simulink model "simulacionfinal"  (R2014a)
settings: Solver=ode3  StartTime=0.0  StopTime=40  FixedStep=0.01  RelTol=1e-12
values from neighbouring files (symbols this model uses):
  m = [1 t0 (t0)^2 (t0)^3;0 1 (2*(t0)^2) (3*(t0)^2);1 tf (tf)^2 (tf)^3;0 1 (2*(tf)^2) (3*(tf)^2)]    [ControlCinematico.m]    (also in untitled3.m = [1 0 0 0 0 0;0 1 0 0 0 0;0 0 2 0 0 0;1 tf tf^2 tf^3 tf^4 tf^)
libraries: mblibv1 x15
settings Model: Creator=sebastian  LastModifiedBy=root
settings DataIOCC: SignalLoggingSaveFormat=ModelDataLogs
settings DebuggingCC: UnderspecifiedInitializationDetection=Classic  MultiTaskDSMMsg=warning  MultiTaskCondExecSysMsg=none  StateNameClashWarn=warning
settings RTWCC: IncludeERTFirstTime=on
settings SimMechanicsCC: VisOnUpdateDiagram=on  VisDuringSimulation=on

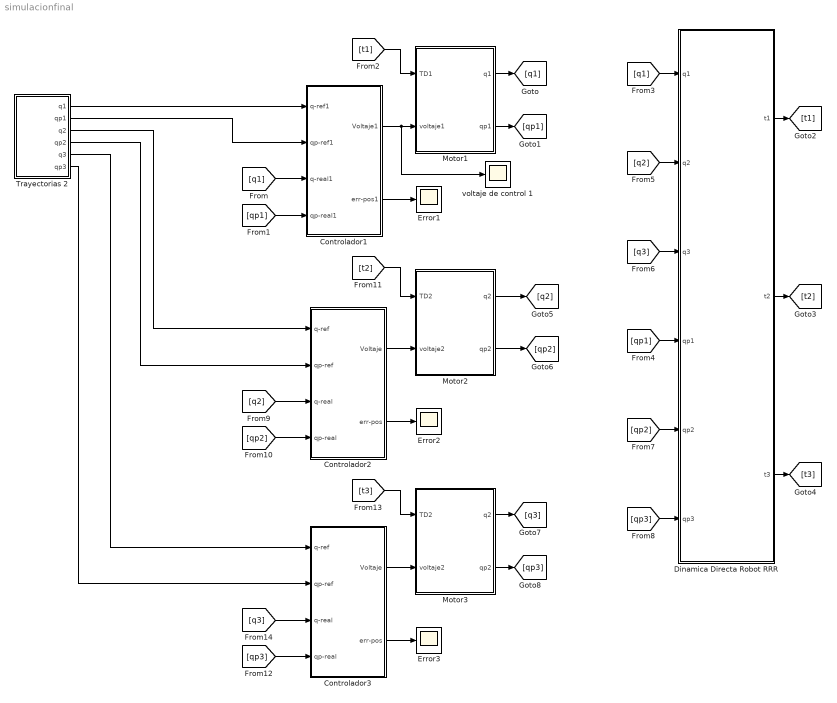
== system simulacionfinal ==
  Controlador1 : Subsystem
  Controlador2 : Subsystem
  Controlador3 : Subsystem
  Dinamica Directa Robot RRR : Subsystem
  Error1 : Scope
      settings: TimeRange=0.000199999999999978  YMin=-470000  YMax=-455000  SaveName=ScopeData4
  Error2 : Scope
      settings: YMin=0.3178  YMax=0.3188
  Error3 : Scope
      settings: YMin=0.675  YMax=1  SaveName=ScopeData5
  Motor1 : Subsystem
  Motor2 : Subsystem
  Motor3 : Subsystem
  Trayectorias 2 : Subsystem
  voltaje de control 1 : Scope
      settings: YMin=-1.5  YMax=1.25  SaveName=ScopeData12
  wires:
  Controlador1/1(Voltaje1) -> voltaje de control 1/1, Motor1/2(voltaje1)
  Controlador1/2(err-pos1) -> Error1/1
  Motor1/1(q1) -> [q1]
  Motor1/2(qp1) -> [qp1]
  Dinamica Directa Robot RRR/1(t1) -> [t1]
  [q1] -> Controlador1/3(q-real1)
  [qp1] -> Controlador1/4(qp-real1)
  [q1] -> Dinamica Directa Robot RRR/1(q1)
  [qp1] -> Dinamica Directa Robot RRR/4(qp1)
  [q2] -> Dinamica Directa Robot RRR/2(q2)
  [q3] -> Dinamica Directa Robot RRR/3(q3)
  [qp2] -> Dinamica Directa Robot RRR/5(qp2)
  [qp3] -> Dinamica Directa Robot RRR/6(qp3)
  Dinamica Directa Robot RRR/2(t2) -> [t2]
  Dinamica Directa Robot RRR/3(t3) -> [t3]
  Controlador2/1(Voltaje) -> Motor2/2(voltaje2)
  Controlador2/2(err-pos) -> Error2/1
  [q2] -> Controlador2/3(q-real)
  [qp2] -> Controlador2/4(qp-real)
  Controlador3/1(Voltaje) -> Motor3/2(voltaje2)
  Controlador3/2(err-pos) -> Error3/1
  Motor3/1(q2) -> [q3]
  Motor3/2(qp2) -> [qp3]
  [q3] -> Controlador3/3(q-real)
  [qp3] -> Controlador3/4(qp-real)
  Motor2/1(q2) -> [q2]
  Motor2/2(qp2) -> [qp2]
  Trayectorias 2/1(q1) -> Controlador1/1(q-ref1)
  Trayectorias 2/2(qp1) -> Controlador1/2(qp-ref1)
  Trayectorias 2/3(q2) -> Controlador2/1(q-ref)
  Trayectorias 2/4(qp2) -> Controlador2/2(qp-ref)
  Trayectorias 2/5(q3) -> Controlador3/1(q-ref)
  Trayectorias 2/6(qp3) -> Controlador3/2(qp-ref)
  [t1] -> Motor1/1(TD1)
  [t2] -> Motor2/1(TD2)
  [t3] -> Motor3/1(TD2)

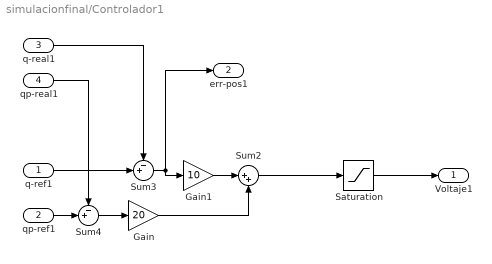
== system simulacionfinal/Controlador1 ==
  q-ref1 : Inport
  qp-ref1 : Inport  Port=2
  q-real1 : Inport  Port=3
  qp-real1 : Inport  Port=4
  Gain : Gain  Gain=20
  Gain1 : Gain  Gain=10
  Saturation : Saturate  UpperLimit=1.5  LowerLimit=-1.5
  Sum2 : Sum  Inputs=|++
  Sum3 : Sum  Inputs=-+|
  Sum4 : Sum  Inputs=-+|
  Voltaje1 : Outport
  err-pos1 : Outport  Port=2
  wires:
  Gain1/1 -> Sum2/1
  Gain/1 -> Sum2/2
  Sum4/1 -> Gain/1
  Sum2/1 -> Saturation/1
  q-ref1/1 -> Sum3/2
  qp-ref1/1 -> Sum4/2
  q-real1/1 -> Sum3/1
  qp-real1/1 -> Sum4/1
  Sum3/1 -> Gain1/1, err-pos1/1
  Saturation/1 -> Voltaje1/1

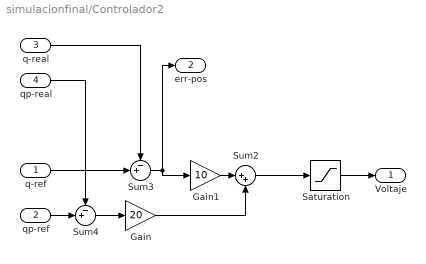
== system simulacionfinal/Controlador2 ==
  q-ref : Inport
  qp-ref : Inport  Port=2
  q-real : Inport  Port=3
  qp-real : Inport  Port=4
  Gain : Gain  Gain=20
  Gain1 : Gain  Gain=10
  Saturation : Saturate  UpperLimit=1.5  LowerLimit=-1.5
  Sum2 : Sum  Inputs=|++
  Sum3 : Sum  Inputs=-+|
  Sum4 : Sum  Inputs=-+|
  Voltaje : Outport
  err-pos : Outport  Port=2
  wires:
  Gain1/1 -> Sum2/1
  Gain/1 -> Sum2/2
  Sum4/1 -> Gain/1
  Sum2/1 -> Saturation/1
  q-ref/1 -> Sum3/2
  qp-ref/1 -> Sum4/2
  q-real/1 -> Sum3/1
  qp-real/1 -> Sum4/1
  Sum3/1 -> Gain1/1, err-pos/1
  Saturation/1 -> Voltaje/1

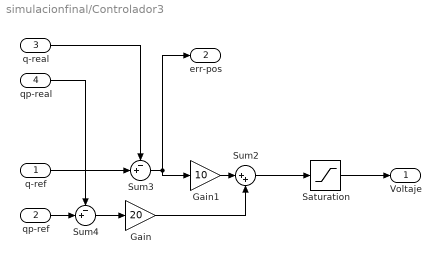
== system simulacionfinal/Controlador3 ==
  q-ref : Inport
  qp-ref : Inport  Port=2
  q-real : Inport  Port=3
  qp-real : Inport  Port=4
  Gain : Gain  Gain=20
  Gain1 : Gain  Gain=10
  Saturation : Saturate  UpperLimit=1.5  LowerLimit=-1.5
  Sum2 : Sum  Inputs=|++
  Sum3 : Sum  Inputs=-+|
  Sum4 : Sum  Inputs=-+|
  Voltaje : Outport
  err-pos : Outport  Port=2
  wires:
  Gain1/1 -> Sum2/1
  Gain/1 -> Sum2/2
  Sum4/1 -> Gain/1
  Sum2/1 -> Saturation/1
  q-ref/1 -> Sum3/2
  qp-ref/1 -> Sum4/2
  q-real/1 -> Sum3/1
  qp-real/1 -> Sum4/1
  Sum3/1 -> Gain1/1, err-pos/1
  Saturation/1 -> Voltaje/1

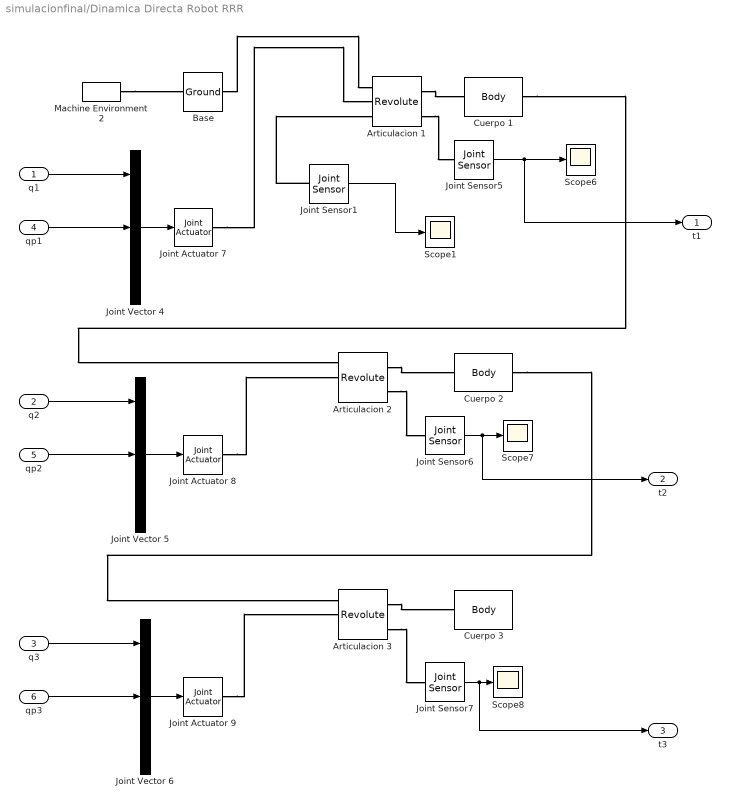
== system simulacionfinal/Dinamica Directa Robot RRR ==
  q1 : Inport
  q2 : Inport  Port=2
  q3 : Inport  Port=3
  qp1 : Inport  Port=4
  qp2 : Inport  Port=5
  qp3 : Inport  Port=6
  Articulacion 1 : mblibv1/Joints/Revolute  LConnTagsString=__newl0|SA1|SA2  RConnTagsString=__newr0|SA1  UpdateFromCAD=off  NumSAPorts=3  CutJoint=off  MarkAsCut=off  Primitives=prismatic  PrimitiveProps=R1$World$[0 0 1]$revolute  DialogClass=JointBlock  R1Axis=[0 0 1]
  Articulacion 2 : mblibv1/Joints/Revolute  LConnTagsString=__newl0|SA1|SA2  RConnTagsString=__newr0|SA1  UpdateFromCAD=off  NumSAPorts=3  CutJoint=off  MarkAsCut=off  Primitives=prismatic  PrimitiveProps=R1$World$[0 0 1]$revolute  DialogClass=JointBlock  R1Axis=[0 0 1]
  Articulacion 3 : mblibv1/Joints/Revolute  LConnTagsString=__newl0|SA1|SA2  RConnTagsString=__newr0|SA1  UpdateFromCAD=off  NumSAPorts=3  CutJoint=off  MarkAsCut=off  Primitives=prismatic  PrimitiveProps=R1$World$[0 0 1]$revolute  DialogClass=JointBlock  R1Axis=[0 0 1]
  Base : mblibv1/Bodies/Ground  UpdateFromCAD=off  LeftPortType=env  RightPortType=workingframe  PhysicalDomain=Mechanical  DialogClass=GroundBlock  CoordPosition=[0 0 0]  CoordPositionUnits=m  StateVectorMgrId=0  MachineId=[1 0]  ShowEnvPort=on  ParameterChecksum=[135980113, 3777956771, 1224883924, 2878565293]  TopologyChecksum=[1058938833, 390769295, 436021046, 484204497]
  Cuerpo 1 : mblibv1/Bodies/Body  LConnTagsString=CS1  RConnTagsString=CS2  UpdateFromCAD=off  DialogClass=MechanicalBodyBlock  Mass=1  MassUnits=kg  InertiaUnits=kg*m^2  Inertia=[0 0 0;0 0 0;0 0 33.3333]  Shape=Cylinder  ShapeDims=[1 1]  ShapeUnits=m  ShapeUse=false  Density=1  DensityUnits=kg/m^3  DensityUse=false  GraphicsMode=MACHINE_DEFAULT  BodyColorSelMode=COLORPALETTE  BodyColor=[0 1 0]  AttachedToCS=CG  CG=Left$CG$[0 10 0]$WORLD$WORLD$m$[0 0 0]$Euler X-Y-Z$deg$WORLD$false$none  WorkingFrames=Left$CS1$[0 0 0]$World$World$m$[0 0 0]$Euler X-Y-Z$deg$WORLD$true$none#Right$CS2$[0 20 0]$World$World$m$[0 0 0]$Euler X-Y-Z$deg$WORLD$true$none  CGPos=[0 10 0]  CGRot=[0 0 0]  CS0Pos=[]  CS0Rot=[]  CS1Pos=[0 0 0]  CS1Rot=[0 0 0]  CS2Pos=[0 20 0]  CS2Rot=[0 0 0]  CS3Pos=[]  CS3Rot=[]  CS4Pos=[]  CS4Rot=[]  CS5Pos=[]  CS5Rot=[]  CS6Pos=[]  CS6Rot=[]  CS7Pos=[]  CS7Rot=[]  CS8Pos=[]  CS8Rot=[]  CS9Pos=[]  CS9Rot=[]  CS10Pos=[]  CS10Rot=[]  CS11Pos=[]  CS11Rot=[]  CS12Pos=[]  CS12Rot=[]  CS13Pos=[]  CS13Rot=[]  CS14Pos=[]  CS14Rot=[]  CS15Pos=[]  CS15Rot=[]  CS16Pos=[]  CS16Rot=[]  CS17Pos=[]  CS17Rot=[]  CS18Pos=[]  CS18Rot=[]  CS19Pos=[]  CS19Rot=[]  CS20Pos=[]  CS20Rot=[]
  Cuerpo 2 : mblibv1/Bodies/Body  LConnTagsString=CS1  RConnTagsString=CS2  UpdateFromCAD=off  DialogClass=MechanicalBodyBlock  Mass=1  MassUnits=kg  InertiaUnits=kg*m^2  Inertia=[0 0 0;0 0 0;0 0 33.3333]  Shape=Cylinder  ShapeDims=[1 1]  ShapeUnits=m  ShapeUse=false  Density=1  DensityUnits=kg/m^3  DensityUse=false  GraphicsMode=MACHINE_DEFAULT  BodyColorSelMode=COLORPALETTE  BodyColor=[0 1 0]  AttachedToCS=CG  CG=Left$CG$[10 20 0]$WORLD$WORLD$m$[0 0 0]$Euler X-Y-Z$deg$WORLD$false$none  WorkingFrames=Left$CS1$[0 20 0]$World$World$m$[0 0 0]$Euler X-Y-Z$deg$WORLD$true$none#Right$CS2$[20 20 0]$World$World$m$[0 0 0]$Euler X-Y-Z$deg$WORLD$true$none  CGPos=[10 20 0]  CGRot=[0 0 0]  CS0Pos=[]  CS0Rot=[]  CS1Pos=[0 20 0]  CS1Rot=[0 0 0]  CS2Pos=[20 20 0]  CS2Rot=[0 0 0]  CS3Pos=[]  CS3Rot=[]  CS4Pos=[]  CS4Rot=[]  CS5Pos=[]  CS5Rot=[]  CS6Pos=[]  CS6Rot=[]  CS7Pos=[]  CS7Rot=[]  CS8Pos=[]  CS8Rot=[]  CS9Pos=[]  CS9Rot=[]  CS10Pos=[]  CS10Rot=[]  CS11Pos=[]  CS11Rot=[]  CS12Pos=[]  CS12Rot=[]  CS13Pos=[]  CS13Rot=[]  CS14Pos=[]  CS14Rot=[]  CS15Pos=[]  CS15Rot=[]  CS16Pos=[]  CS16Rot=[]  CS17Pos=[]  CS17Rot=[]  CS18Pos=[]  CS18Rot=[]  CS19Pos=[]  CS19Rot=[]  CS20Pos=[]  CS20Rot=[]
  Cuerpo 3 : mblibv1/Bodies/Body  LConnTagsString=CS1  RConnTagsString=CS2  UpdateFromCAD=off  DialogClass=MechanicalBodyBlock  Mass=1  MassUnits=kg  InertiaUnits=kg*m^2  Inertia=[0 0 0;0 0 0;0 0 8.3333]  Shape=Cylinder  ShapeDims=[1 1]  ShapeUnits=m  ShapeUse=false  Density=1  DensityUnits=kg/m^3  DensityUse=false  GraphicsMode=MACHINE_DEFAULT  BodyColorSelMode=COLORPALETTE  BodyColor=[0 1 0]  AttachedToCS=CG  CG=Left$CG$[20 15 0]$WORLD$WORLD$m$[0 0 0]$Euler X-Y-Z$deg$WORLD$false$none  WorkingFrames=Left$CS1$[20 20 0]$World$World$m$[0 0 0]$Euler X-Y-Z$deg$WORLD$true$none#Right$CS2$[20 10 0]$World$World$m$[0 0 0]$Euler X-Y-Z$deg$WORLD$true$none  CGPos=[20 15 0]  CGRot=[0 0 0]  CS0Pos=[]  CS0Rot=[]  CS1Pos=[20 20 0]  CS1Rot=[0 0 0]  CS2Pos=[20 10 0]  CS2Rot=[0 0 0]  CS3Pos=[]  CS3Rot=[]  CS4Pos=[]  CS4Rot=[]  CS5Pos=[]  CS5Rot=[]  CS6Pos=[]  CS6Rot=[]  CS7Pos=[]  CS7Rot=[]  CS8Pos=[]  CS8Rot=[]  CS9Pos=[]  CS9Rot=[]  CS10Pos=[]  CS10Rot=[]  CS11Pos=[]  CS11Rot=[]  CS12Pos=[]  CS12Rot=[]  CS13Pos=[]  CS13Rot=[]  CS14Pos=[]  CS14Rot=[]  CS15Pos=[]  CS15Rot=[]  CS16Pos=[]  CS16Rot=[]  CS17Pos=[]  CS17Rot=[]  CS18Pos=[]  CS18Rot=[]  CS19Pos=[]  CS19Rot=[]  CS20Pos=[]  CS20Rot=[]
  Joint Actuator 7 : mblibv1/Sensors &  Actuators/Joint Actuator  UpdateFromCAD=off  PhysicalDomain=Mechanical  PortType=blob  ActuationStyle=Motion  AngleUnits=rad  ArcVelocityUnits=rad/s  ArcAccelerationUnits=rad/s^2  CoordPositionUnits=m  VelocityUnits=m/s  AccelerationUnits=m/s^2  ForceUnits=N  TorqueUnits=N*m  ActiveIO=on  Width=3  DialogClass=MechanicalActuatorBlock  Primitive=R1  ReferenceFrame=Absolute (World)
  Joint Actuator 8 : mblibv1/Sensors &  Actuators/Joint Actuator  UpdateFromCAD=off  PhysicalDomain=Mechanical  PortType=blob  ActuationStyle=Motion  AngleUnits=rad  ArcVelocityUnits=rad/s  ArcAccelerationUnits=rad/s^2  CoordPositionUnits=m  VelocityUnits=m/s  AccelerationUnits=m/s^2  ForceUnits=N  TorqueUnits=N*m  ActiveIO=on  Width=3  DialogClass=MechanicalActuatorBlock  Primitive=R1  ReferenceFrame=Absolute (World)
  Joint Actuator 9 : mblibv1/Sensors &  Actuators/Joint Actuator  UpdateFromCAD=off  PhysicalDomain=Mechanical  PortType=blob  ActuationStyle=Motion  AngleUnits=rad  ArcVelocityUnits=rad/s  ArcAccelerationUnits=rad/s^2  CoordPositionUnits=m  VelocityUnits=m/s  AccelerationUnits=m/s^2  ForceUnits=N  TorqueUnits=N*m  ActiveIO=on  Width=3  DialogClass=MechanicalActuatorBlock  Primitive=R1  ReferenceFrame=Absolute (World)
  Joint Sensor1 : mblibv1/Sensors &  Actuators/Joint Sensor  UpdateFromCAD=off  PhysicalDomain=Mechanical  PortType=blob  Muxed=on  Pose=off  Angle=on  AngleUnits=rad  ArcVelocity=off  ArcVelocityUnits=deg/s  ArcAcceleration=off  ArcAccelerationUnits=deg/s^2  CoordPosition=on  CoordPositionUnits=m  Velocity=off  VelocityUnits=m/s  Acceleration=off  AccelerationUnits=m/s^2  Quaternion=on  QuaternionDT=off  QuaternionDDT=off  QuaternionUnits=off  OutputVector=[1]  ActiveIO=on  Width=1  DialogClass=MechanicalSensorBlock  Primitive=R1  Force=off  ForceUnits=N  Torque=off  TorqueUnits=N*m  ReferenceFrame=Absolute (World)  ReactionSensedSide=Follower  ReactionReferenceFrame=Absolute (World)  ReactionForce=off  ReactionForceUnits=N  ReactionMoment=off  ReactionMomentUnits=N*m
  Joint Sensor5 : mblibv1/Sensors &  Actuators/Joint Sensor  UpdateFromCAD=off  PhysicalDomain=Mechanical  PortType=blob  Muxed=on  Pose=off  Angle=off  AngleUnits=deg  ArcVelocity=off  ArcVelocityUnits=deg/s  ArcAcceleration=off  ArcAccelerationUnits=deg/s^2  CoordPosition=on  CoordPositionUnits=m  Velocity=off  VelocityUnits=m/s  Acceleration=off  AccelerationUnits=m/s^2  Quaternion=on  QuaternionDT=off  QuaternionDDT=off  QuaternionUnits=off  OutputVector=[1]  ActiveIO=on  Width=1  DialogClass=MechanicalSensorBlock  Primitive=R1  Force=off  ForceUnits=N  Torque=on  TorqueUnits=N*m  ReferenceFrame=Absolute (World)  ReactionSensedSide=Follower  ReactionReferenceFrame=Absolute (World)  ReactionForce=off  ReactionForceUnits=N  ReactionMoment=off  ReactionMomentUnits=N*m
  Joint Sensor6 : mblibv1/Sensors &  Actuators/Joint Sensor  UpdateFromCAD=off  PhysicalDomain=Mechanical  PortType=blob  Muxed=on  Pose=off  Angle=off  AngleUnits=deg  ArcVelocity=off  ArcVelocityUnits=deg/s  ArcAcceleration=off  ArcAccelerationUnits=deg/s^2  CoordPosition=on  CoordPositionUnits=m  Velocity=off  VelocityUnits=m/s  Acceleration=off  AccelerationUnits=m/s^2  Quaternion=on  QuaternionDT=off  QuaternionDDT=off  QuaternionUnits=off  OutputVector=[1]  ActiveIO=on  Width=1  DialogClass=MechanicalSensorBlock  Primitive=R1  Force=off  ForceUnits=N  Torque=on  TorqueUnits=N*m  ReferenceFrame=Absolute (World)  ReactionSensedSide=Follower  ReactionReferenceFrame=Absolute (World)  ReactionForce=off  ReactionForceUnits=N  ReactionMoment=off  ReactionMomentUnits=N*m
  Joint Sensor7 : mblibv1/Sensors &  Actuators/Joint Sensor  UpdateFromCAD=off  PhysicalDomain=Mechanical  PortType=blob  Muxed=on  Pose=off  Angle=off  AngleUnits=deg  ArcVelocity=off  ArcVelocityUnits=deg/s  ArcAcceleration=off  ArcAccelerationUnits=deg/s^2  CoordPosition=on  CoordPositionUnits=m  Velocity=off  VelocityUnits=m/s  Acceleration=off  AccelerationUnits=m/s^2  Quaternion=on  QuaternionDT=off  QuaternionDDT=off  QuaternionUnits=off  OutputVector=[1]  ActiveIO=on  Width=1  DialogClass=MechanicalSensorBlock  Primitive=R1  Force=off  ForceUnits=N  Torque=on  TorqueUnits=N*m  ReferenceFrame=Absolute (World)  ReactionSensedSide=Follower  ReactionReferenceFrame=Absolute (World)  ReactionForce=off  ReactionForceUnits=N  ReactionMoment=off  ReactionMomentUnits=N*m
  Joint Vector 4 : Concatenate  NumInputs=3
  Joint Vector 5 : Concatenate  NumInputs=3
  Joint Vector 6 : Concatenate  NumInputs=3
  Machine Environment2 : mblibv1/Bodies/Machine Environment  PortType=env  PhysicalDomain=Mechanical  DialogTemplateClass=MECH.MachineEnvironment  SyncWhenCopied=off  Gravity=[0 0 0]  GravityUnits=m/s^2  GravityAsSignal=off  Dimensionality=Auto-detect  AnalysisType=Inverse dynamics  LinearAssemblyTolerance=1e-3  LinearAssemblyToleranceUnits=m  AngularAssemblyTolerance=1e-3  AngularAssemblyToleranceUnits=rad  ConstraintSolverType=Stabilizing  ConstraintRelTolerance=1e-4  ConstraintAbsTolerance=1e-4  UseRobustSingularityHandling=off  RedundancyAnalysisToleranceType=Automatically select tolerance  RedundancyAnalysisTolerance=1e-14  StatePerturbationType=Fixed  PerturbationSize=1e-5  VisualizeMachine=on  BodyVisualizationType=Use model default body geometries  BodyColorSelMode=Use model default  DefaultBodyColor=[1 0 0]
  Scope{1,6..8} (4 alike) : Scope
      Scope1 settings: TimeRange=30  YMin=-2.525e+08  YMax=-2.35e+08  SaveName=ScopeData13
      Scope6 settings: TimeRange=30  YMin=-2.525e+08  YMax=-2.35e+08  SaveName=ScopeData9
      Scope7 settings: TimeRange=30  SaveName=ScopeData10
      Scope8 settings: TimeRange=30  SaveName=ScopeData11
  t1 : Outport
  t2 : Outport  Port=2
  t3 : Outport  Port=3
  wires:
  Joint Vector 5/1 -> Joint Actuator 8/1
  Joint Vector 4/1 -> Joint Actuator 7/1
  Joint Vector 6/1 -> Joint Actuator 9/1
  Joint Sensor5/1 -> t1/1, Scope6/1
  Joint Sensor7/1 -> t3/1, Scope8/1
  Joint Sensor6/1 -> t2/1, Scope7/1
  q1/1 -> Joint Vector 4/1
  q2/1 -> Joint Vector 5/1
  q3/1 -> Joint Vector 6/1
  qp1/1 -> Joint Vector 4/2
  qp2/1 -> Joint Vector 5/2
  qp3/1 -> Joint Vector 6/2
  Joint Sensor1/1 -> Scope1/1
  connections:
  Articulacion 3/RConn1 -- Cuerpo 3/LConn1
  Cuerpo 1/RConn1 -- Articulacion 2/LConn1
  Cuerpo 2/RConn1 -- Articulacion 3/LConn1
  Articulacion 2/RConn2 -- Joint Sensor6/LConn1
  Joint Actuator 8/RConn1 -- Articulacion 2/LConn2
  Articulacion 2/RConn1 -- Cuerpo 2/LConn1
  Base/RConn1 -- Articulacion 1/LConn1
  Articulacion 1/RConn1 -- Cuerpo 1/LConn1
  Articulacion 1/RConn2 -- Joint Sensor5/LConn1
  Articulacion 3/RConn2 -- Joint Sensor7/LConn1
  Joint Actuator 9/RConn1 -- Articulacion 3/LConn2
  Machine Environment2/RConn1 -- Base/LConn1
  Joint Actuator 7/RConn1 -- Articulacion 1/LConn2
  Joint Sensor1/LConn1 -- Articulacion 1/LConn3

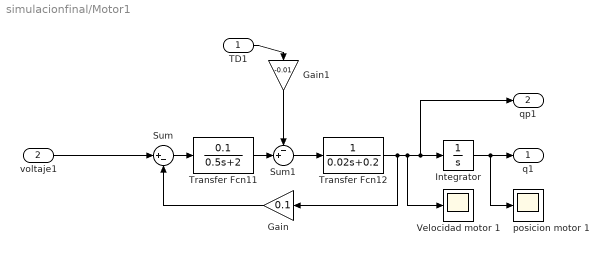
== system simulacionfinal/Motor1 ==
  TD1 : Inport
  voltaje1 : Inport  Port=2
  Gain : Gain  Gain=0.1
  Gain1 : Gain  Gain=-0.01
  Integrator : Integrator
  Sum : Sum  Inputs=|+-
  Sum1 : Sum  Inputs=-+|
  Transfer Fcn11 : TransferFcn  Numerator=[0.1]  Denominator=[0.5 2]
  Transfer Fcn12 : TransferFcn  Denominator=[0.02 0.2]
  Velocidad motor 1 : Scope
  posicion motor 1 : Scope
      settings: SaveName=ScopeData3
  q1 : Outport
  qp1 : Outport  Port=2
  wires:
  Sum/1 -> Transfer Fcn11/1
  Sum1/1 -> Transfer Fcn12/1
  Transfer Fcn11/1 -> Sum1/2
  Gain/1 -> Sum/2
  Transfer Fcn12/1 -> qp1/1, Integrator/1, Velocidad motor 1/1, Gain/1
  Integrator/1 -> q1/1, posicion motor 1/1
  voltaje1/1 -> Sum/1
  TD1/1 -> Gain1/1
  Gain1/1 -> Sum1/1

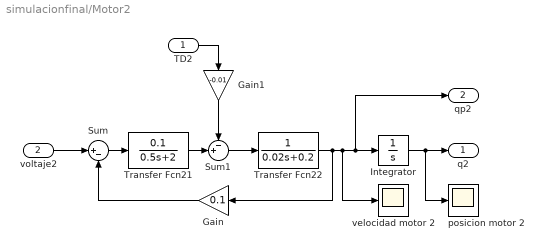
== system simulacionfinal/Motor2 ==
  TD2 : Inport
  voltaje2 : Inport  Port=2
  Gain : Gain  Gain=0.1
  Gain1 : Gain  Gain=-0.01
  Integrator : Integrator
  Sum : Sum  Inputs=|+-
  Sum1 : Sum  Inputs=-+|
  Transfer Fcn21 : TransferFcn  Numerator=[0.1]  Denominator=[0.5 2]
  Transfer Fcn22 : TransferFcn  Denominator=[0.02 0.2]
  posicion motor 2 : Scope
      settings: SaveName=ScopeData3
  velocidad motor 2 : Scope
  q2 : Outport
  qp2 : Outport  Port=2
  wires:
  Sum/1 -> Transfer Fcn21/1
  Sum1/1 -> Transfer Fcn22/1
  Transfer Fcn21/1 -> Sum1/2
  Gain/1 -> Sum/2
  Transfer Fcn22/1 -> qp2/1, Integrator/1, velocidad motor 2/1, Gain/1
  Integrator/1 -> q2/1, posicion motor 2/1
  voltaje2/1 -> Sum/1
  TD2/1 -> Gain1/1
  Gain1/1 -> Sum1/1

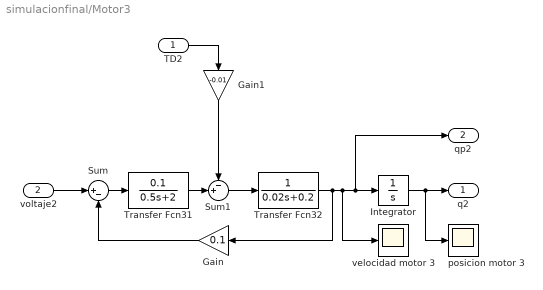
== system simulacionfinal/Motor3 ==
  TD2 : Inport
  voltaje2 : Inport  Port=2
  Gain : Gain  Gain=0.1
  Gain1 : Gain  Gain=-0.01
  Integrator : Integrator
  Sum : Sum  Inputs=|+-
  Sum1 : Sum  Inputs=-+|
  Transfer Fcn31 : TransferFcn  Numerator=[0.1]  Denominator=[0.5 2]
  Transfer Fcn32 : TransferFcn  Denominator=[0.02 0.2]
  posicion motor 3 : Scope
      settings: SaveName=ScopeData3
  velocidad motor 3 : Scope
  q2 : Outport
  qp2 : Outport  Port=2
  wires:
  Sum/1 -> Transfer Fcn31/1
  Sum1/1 -> Transfer Fcn32/1
  Transfer Fcn31/1 -> Sum1/2
  Gain/1 -> Sum/2
  Transfer Fcn32/1 -> qp2/1, Integrator/1, velocidad motor 3/1, Gain/1
  Integrator/1 -> q2/1, posicion motor 3/1
  voltaje2/1 -> Sum/1
  TD2/1 -> Gain1/1
  Gain1/1 -> Sum1/1

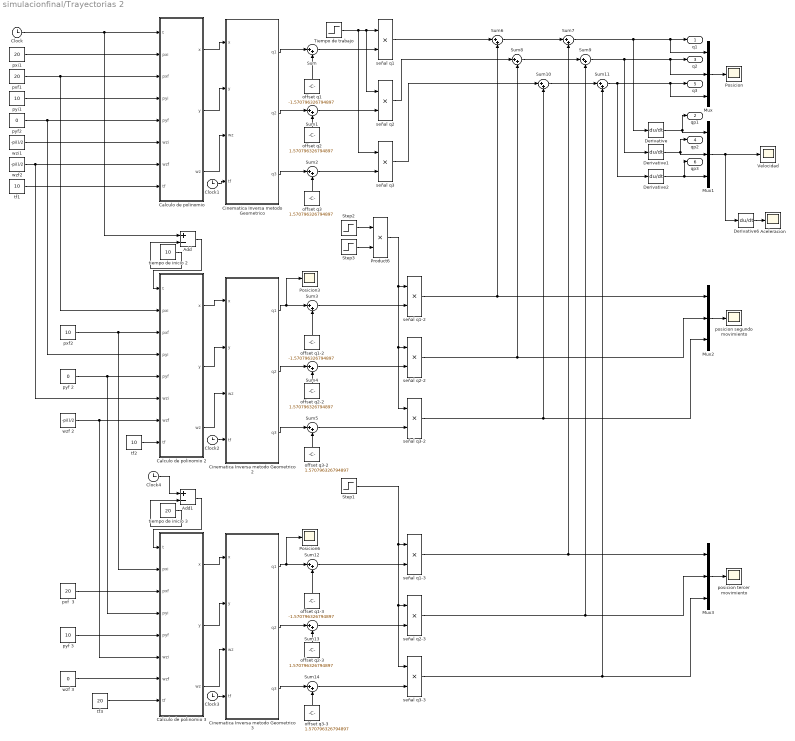
== system simulacionfinal/Trayectorias 2 ==
  Aceleracion : Scope
      settings: TimeRange=40  SaveName=ScopeData29
  Add : Sum  Inputs=+-
  Add1 : Sum  Inputs=+-
  Calculo de polinomio : MATLAB Function  TreatAsAtomicUnit=on
  Calculo de polinomio 2 : MATLAB Function  TreatAsAtomicUnit=on
  Calculo de polinomio 3 : MATLAB Function  TreatAsAtomicUnit=on
  "Cinematica Inversa metodo Geometrico " : MATLAB Function  TreatAsAtomicUnit=on
  Cinematica Inversa metodo Geometrico 2 : MATLAB Function  TreatAsAtomicUnit=on
  Cinematica Inversa metodo Geometrico 3 : MATLAB Function  TreatAsAtomicUnit=on
  Clock{,1..4} (5 alike) : Clock
  Derivative{,1..2,6} (4 alike) : Derivative
  Mux{,1..3} (4 alike) : Mux  Inputs=3
  Posicion : Scope
      settings: TimeRange=1.736204576043068  YMin=-0.9624756335282649  YMax=0.6817738791423005  SaveName=ScopeData14
  Posicion3 : Scope
      settings: YMin=1.25221  YMax=1.38403  SaveName=ScopeData18
  Posicion6 : Scope
      settings: SaveName=ScopeData21
  Product6 : Product
  Step1 : Step  Time=20  SampleTime=0
  Step2 : Step  Time=10  SampleTime=0
  Step3 : Step  Time=20  Before=1  After=0  SampleTime=0
  Sum{,1..14} (15 alike) : Sum  Inputs=|++
  Tiempo de trabajo : Step  Time=10  Before=1  After=0  SampleTime=0
  Velocidad : Scope
      settings: TimeRange=40  SaveName=ScopeData15
  offset q1 : Constant  Value=-1.570796326794897
  offset q1-2 : Constant  Value=-1.570796326794897
  offset q1-3 : Constant  Value=-1.570796326794897
  offset q2 : Constant  Value=1.570796326794897
  offset q2-2 : Constant  Value=1.570796326794897
  offset q2-3 : Constant  Value=1.570796326794897
  offset q3 : Constant  Value=1.570796326794897
  offset q3-2 : Constant  Value=1.570796326794897
  offset q3-3 : Constant  Value=1.570796326794897
  posicion segundo movimiento : Scope
      settings: SaveName=ScopeData16
  posicion tercer movimiento : Scope
      settings: SaveName=ScopeData20
  pxf  3 : Constant  Value=20
  pxf1 : Constant  Value=20
  pxf2 : Constant  Value=10
  pxi1 : Constant  Value=20
  pyf 2 : Constant  Value=0
  pyf 3 : Constant  Value=10
  pyf2 : Constant  Value=0
  pyi1 : Constant  Value=10
  señal q1 : Product
  señal q1-2 : Product
  señal q1-3 : Product
  señal q2 : Product
  señal q2-2 : Product
  señal q2-3 : Product
  señal q3 : Product
  señal q3-2 : Product
  señal q3-3 : Product
  tf1 : Constant  Value=10
  tf2 : Constant  Value=10
  tf3 : Constant  Value=20
  tiempo de inicio 2 : Constant  Value=10
  tiempo de inicio 3 : Constant  Value=20
  wzf 2 : Constant  Value=-pi()/2
  wzf 3 : Constant  Value=0
  wzf2 : Constant  Value=-pi()/2
  wzi1 : Constant  Value=-pi()/2
  q1 : Outport
  qp1 : Outport  Port=2
  q2 : Outport  Port=3
  qp2 : Outport  Port=4
  q3 : Outport  Port=5
  qp3 : Outport  Port=6
  wires:
  Mux/1 -> Posicion/1
  Mux1/1 -> Derivative6/1, Velocidad/1
  Derivative/1 -> Mux1/1, qp1/1
  Derivative2/1 -> qp3/1, Mux1/3
  Derivative1/1 -> Mux1/2, qp2/1
  pxi1/1 -> Calculo de polinomio/2(pxi)
  pyi1/1 -> Calculo de polinomio/4(pyi)
  tf1/1 -> Calculo de polinomio/8(tf)
  Calculo de polinomio/3(wz) -> "Cinematica Inversa metodo Geometrico "/3(wz)
  Calculo de polinomio/1(x) -> "Cinematica Inversa metodo Geometrico "/1(x)
  Calculo de polinomio/2(y) -> "Cinematica Inversa metodo Geometrico "/2(y)
  wzi1/1 -> Calculo de polinomio/6(wzi)
  "Cinematica Inversa metodo Geometrico "/2(q2) -> Sum1/1
  "Cinematica Inversa metodo Geometrico "/3(q3) -> Sum2/1
  offset q2/1 -> Sum1/2
  offset q1/1 -> Sum/2
  "Cinematica Inversa metodo Geometrico "/1(q1) -> Sum/1
  offset q3/1 -> Sum2/2
  Clock/1 -> Calculo de polinomio/1(t), Add/1
  pxf1/1 -> Calculo de polinomio 2/2(pxi), Calculo de polinomio/3(pxf)
  pyf2/1 -> Calculo de polinomio 2/4(pyi), Calculo de polinomio/5(pyf)
  pyf 2/1 -> Calculo de polinomio 3/4(pyi), Calculo de polinomio 2/5(pyf)
  wzf 2/1 -> Calculo de polinomio 3/6(wzi), Calculo de polinomio 2/7(wzf)
  tf2/1 -> Calculo de polinomio 2/8(tf)
  wzf2/1 -> Calculo de polinomio 2/6(wzi), Calculo de polinomio/7(wzf)
  Tiempo de trabajo/1 -> señal q3/1, señal q2/1, señal q1/1
  Cinematica Inversa metodo Geometrico 2/2(q2) -> Sum4/1
  Cinematica Inversa metodo Geometrico 2/3(q3) -> Sum5/1
  offset q2-2/1 -> Sum4/2
  offset q1-2/1 -> Sum3/2
  Cinematica Inversa metodo Geometrico 2/1(q1) -> Posicion3/1, Sum3/1
  offset q3-2/1 -> Sum5/2
  Sum2/1 -> señal q3/2
  Sum1/1 -> señal q2/2
  Sum/1 -> señal q1/2
  Sum6/1 -> Sum7/1
  Sum7/1 -> Mux/1, q1/1, Derivative/1
  Sum8/1 -> Sum9/1
  Sum9/1 -> Mux/2, q2/1, Derivative1/1
  Sum10/1 -> Sum11/1
  Sum11/1 -> Mux/3, q3/1, Derivative2/1
  señal q1/1 -> Sum6/1
  señal q2/1 -> Sum8/1
  señal q3/1 -> Sum10/1
  Sum3/1 -> señal q1-2/2
  Sum4/1 -> señal q2-2/2
  Sum5/1 -> señal q3-2/2
  Mux2/1 -> posicion segundo movimiento/1
  señal q2-2/1 -> Sum8/2, Mux2/2
  señal q3-2/1 -> Sum10/2, Mux2/3
  Add/1 -> Calculo de polinomio 2/1(t)
  tiempo de inicio 2/1 -> Add/2
  Step2/1 -> Product6/1
  Step3/1 -> Product6/2
  Product6/1 -> señal q3-2/1, señal q2-2/1, señal q1-2/1
  pxf  3/1 -> Calculo de polinomio 3/3(pxf)
  pyf 3/1 -> Calculo de polinomio 3/5(pyf)
  wzf 3/1 -> Calculo de polinomio 3/7(wzf)
  tf3/1 -> Calculo de polinomio 3/8(tf)
  Calculo de polinomio 3/3(wz) -> Cinematica Inversa metodo Geometrico 3/3(wz)
  Calculo de polinomio 3/1(x) -> Cinematica Inversa metodo Geometrico 3/1(x)
  Calculo de polinomio 3/2(y) -> Cinematica Inversa metodo Geometrico 3/2(y)
  Cinematica Inversa metodo Geometrico 3/2(q2) -> Sum13/1
  Cinematica Inversa metodo Geometrico 3/3(q3) -> Sum14/1
  offset q2-3/1 -> Sum13/2
  offset q1-3/1 -> Sum12/2
  Cinematica Inversa metodo Geometrico 3/1(q1) -> Posicion6/1, Sum12/1
  offset q3-3/1 -> Sum14/2
  Sum12/1 -> señal q1-3/2
  Sum13/1 -> señal q2-3/2
  Sum14/1 -> señal q3-3/2
  Mux3/1 -> posicion tercer movimiento/1
  señal q2-3/1 -> Sum9/2, Mux3/2
  señal q3-3/1 -> Mux3/3, Sum11/2
  Add1/1 -> Calculo de polinomio 3/1(t)
  tiempo de inicio 3/1 -> Add1/2
  Step1/1 -> señal q3-3/1, señal q2-3/1, señal q1-3/1
  pxf2/1 -> Calculo de polinomio 3/2(pxi), Calculo de polinomio 2/3(pxf)
  Clock4/1 -> Add1/1
  Calculo de polinomio 2/1(x) -> Cinematica Inversa metodo Geometrico 2/1(x)
  Calculo de polinomio 2/2(y) -> Cinematica Inversa metodo Geometrico 2/2(y)
  Calculo de polinomio 2/3(wz) -> Cinematica Inversa metodo Geometrico 2/3(wz)
  señal q1-2/1 -> Sum6/2, Mux2/1
  señal q1-3/1 -> Sum7/2, Mux3/1
  Derivative6/1 -> Aceleracion/1
  Clock1/1 -> "Cinematica Inversa metodo Geometrico "/4(tf)
  Clock2/1 -> Cinematica Inversa metodo Geometrico 2/4(tf)
  Clock3/1 -> Cinematica Inversa metodo Geometrico 3/4(tf)

== matlab function simulacionfinal/Trayectorias 2/Cinematica Inversa metodo Geometrico  ==
  data: x input; y input; wz input; q1 output; q2 output; q3 output; tf input
function [q1,q2,q3]= fcn(x,y,wz,tf)
l3=10;
l1=20;
l2=20;

    if tf > 10
    q1=0;
    q2=0;
    q3=0;
    else
xw = x-l3*cos(wz);
yw = y-l3*sin(wz);

q2 = -acos((xw^2 + yw^2 - l1^2 - l2^2)/(2*l1*l2));
q1 = asin((l2*sin(-q2))/(sqrt(xw^2 + yw^2))) + atan(yw/xw);

q3= wz-q1-q2;

    end

== matlab function simulacionfinal/Trayectorias 2/Calculo de polinomio ==
  data: t input; x output; pxi input; pxf input; pyi input; pyf input; wzi input; wzf input; y output; wz output; tf input
function [x,y,wz]= fcn(t,pxi,pxf,pyi,pyf,wzi,wzf,tf)

a0x = pxi;
a1x = 0; %velocidad inicial
a2x = 0; %aceleracion inicial
a3x = (10*(pxf-pxi))/tf^3;
a4x = -(15*(pxf-pxi))/tf^4;
a5x = (6*(pxf-pxi))/tf^5;
x = a0x + a1x*t + a2x*t^2 + a3x*t^3 + a4x*t^4 + a5x*t^5;
a0y = pyi;
a1y = 0; %velocidad inicial
a2y = 0; %aceleracion inicial
a3y = (10*(pyf-pyi))/tf^3;
a4y = -(15*(pyf-pyi))/tf^4;
a5y = (6*(pyf-pyi))/tf^5;
y = a0y + a1y*t + a2y*t^2 + a3y*t^3 + a4y*t^4 + a5y*t^5;
a0wz = wzi;
a1wz = 0; %velocidad inicial
a2wz = 0; %aceleracion inicial
a3wz = (10*(wzf-wzi))/tf^3;
a4wz = -(15*(wzf-wzi))/tf^4;
a5wz = (6*(wzf-wzi))/tf^5;
wz = a0wz + a1wz*t + a2wz*t^2 + a3wz*t^3 + a4wz*t^4 + a5wz*t^5;

== matlab function simulacionfinal/Trayectorias 2/Cinematica Inversa metodo Geometrico 2 ==
  data: x input; y input; wz input; q1 output; q2 output; q3 output; tf input
function [q1,q2,q3]= fcn(x,y,wz,tf)
l3=10;
l1=20;
l2=20;

    if tf < 10
    q1=0;
    q2=0;
    q3=0;
    
    elseif tf > 20
     q1=0;
    q2=0;
    q3=0;
        
    else
        
    xw = x-l3*cos(wz);
    yw = y-l3*sin(wz);

    q2 = -acos((xw^2 + yw^2 - l1^2 - l2^2)/(2*l1*l2));
    q1 = asin((l2*sin(-q2))/(sqrt(xw^2 + yw^2))) + atan(yw/xw);

    q3= wz-q1-q2;

    end

== matlab function simulacionfinal/Trayectorias 2/Calculo de polinomio 2 ==
  data: t input; x output; pxi input; pxf input; pyi input; pyf input; wzi input; wzf input; y output; wz output; tf input
function [x,y,wz]= fcn(t,pxi,pxf,pyi,pyf,wzi,wzf,tf)

a0x = pxi;
a1x = 0; %velocidad inicial
a2x = 0; %aceleracion inicial
a3x = (10*(pxf-pxi))/tf^3;
a4x = -(15*(pxf-pxi))/tf^4;
a5x = (6*(pxf-pxi))/tf^5;
x = a0x + a1x*t + a2x*t^2 + a3x*t^3 + a4x*t^4 + a5x*t^5;
a0y = pyi;
a1y = 0; %velocidad inicial
a2y = 0; %aceleracion inicial
a3y = (10*(pyf-pyi))/tf^3;
a4y = -(15*(pyf-pyi))/tf^4;
a5y = (6*(pyf-pyi))/tf^5;
y = a0y + a1y*t + a2y*t^2 + a3y*t^3 + a4y*t^4 + a5y*t^5;
a0wz = wzi;
a1wz = 0; %velocidad inicial
a2wz = 0; %aceleracion inicial
a3wz = (10*(wzf-wzi))/tf^3;
a4wz = -(15*(wzf-wzi))/tf^4;
a5wz = (6*(wzf-wzi))/tf^5;
wz = a0wz + a1wz*t + a2wz*t^2 + a3wz*t^3 + a4wz*t^4 + a5wz*t^5;

== matlab function simulacionfinal/Trayectorias 2/Cinematica Inversa metodo Geometrico 3 ==
  data: x input; y input; wz input; q1 output; q2 output; q3 output; tf input
function [q1,q2,q3]= fcn(x,y,wz,tf)
l3=10;
l1=20;
l2=20;

    if tf < 20
    q1=0;
    q2=0;
    q3=0;
    
    elseif tf > 40
     q1=0;
    q2=0;
    q3=0;
        
    else
        
    xw = x-l3*cos(wz);
    yw = y-l3*sin(wz);

    q2 = -acos((xw^2 + yw^2 - l1^2 - l2^2)/(2*l1*l2));
    q1 = asin((l2*sin(-q2))/(sqrt(xw^2 + yw^2))) + atan(yw/xw);

    q3= wz-q1-q2;

    end

== matlab function simulacionfinal/Trayectorias 2/Calculo de polinomio 3 ==
  data: t input; x output; pxi input; pxf input; pyi input; pyf input; wzi input; wzf input; y output; wz output; tf input
function [x,y,wz]= fcn(t,pxi,pxf,pyi,pyf,wzi,wzf,tf)

a0x = pxi;
a1x = 0; %velocidad inicial
a2x = 0; %aceleracion inicial
a3x = (10*(pxf-pxi))/tf^3;
a4x = -(15*(pxf-pxi))/tf^4;
a5x = (6*(pxf-pxi))/tf^5;
x = a0x + a1x*t + a2x*t^2 + a3x*t^3 + a4x*t^4 + a5x*t^5;
a0y = pyi;
a1y = 0; %velocidad inicial
a2y = 0; %aceleracion inicial
a3y = (10*(pyf-pyi))/tf^3;
a4y = -(15*(pyf-pyi))/tf^4;
a5y = (6*(pyf-pyi))/tf^5;
y = a0y + a1y*t + a2y*t^2 + a3y*t^3 + a4y*t^4 + a5y*t^5;
a0wz = wzi;
a1wz = 0; %velocidad inicial
a2wz = 0; %aceleracion inicial
a3wz = (10*(wzf-wzi))/tf^3;
a4wz = -(15*(wzf-wzi))/tf^4;
a5wz = (6*(wzf-wzi))/tf^5;
wz = a0wz + a1wz*t + a2wz*t^2 + a3wz*t^3 + a4wz*t^4 + a5wz*t^5;
